simulink model "lookuptable3D"  (Simulink 7.8)
settings: Solver=FixedStepDiscrete  StartTime=0.0  StopTime=10.0  FixedStep=1  RelTol=1e-3
settings Model: Creator=hnine  LastModifiedBy=meta
settings GRTTargetCC: CombineOutputUpdateFcns=on

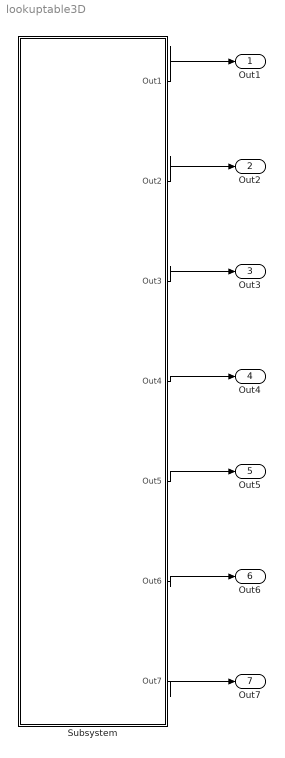
== system lookuptable3D ==
  Subsystem : Subsystem
  Out1 : Outport
  Out2 : Outport  Port=2
  Out3 : Outport  Port=3
  Out4 : Outport  Port=4
  Out5 : Outport  Port=5
  Out6 : Outport  Port=6
  Out7 : Outport  Port=7
  wires:
  Subsystem/1(Out1) -> Out1/1
  Subsystem/2(Out2) -> Out2/1
  Subsystem/3(Out3) -> Out3/1
  Subsystem/7(Out7) -> Out7/1
  Subsystem/4(Out4) -> Out4/1
  Subsystem/5(Out5) -> Out5/1
  Subsystem/6(Out6) -> Out6/1

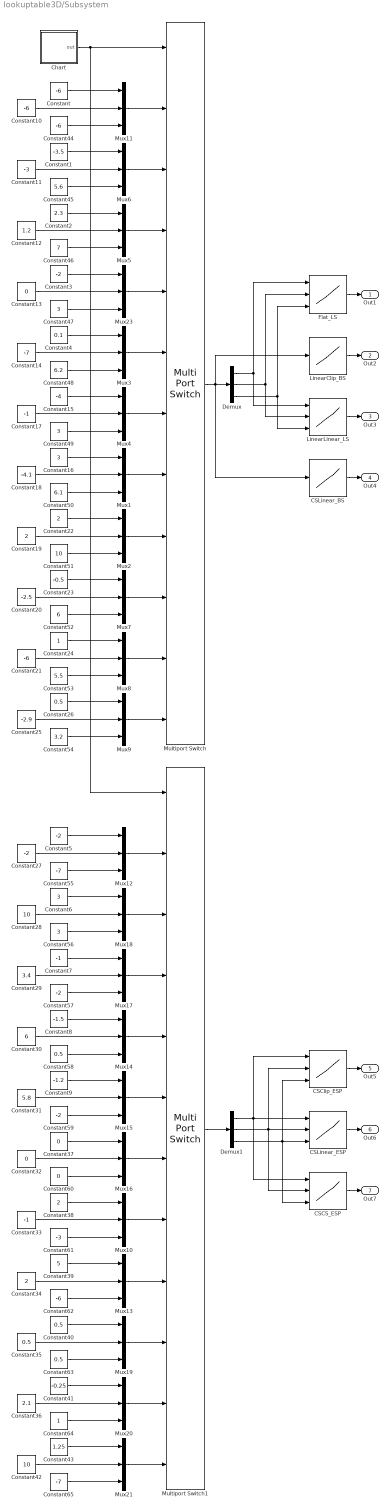
== system lookuptable3D/Subsystem ==
  CSCS_ESP : Lookup_n-D  NumberOfTableDimensions=3  BreakpointsForDimension1=[ -1.5 -0.5 0.5 1.5 ]  BreakpointsForDimension2=[ 0 3 6 9 ]  BreakpointsForDimension3=[ -4 -2.5 -1 0.5 ]  IndexSearchMethod=Evenly spaced points  Table=reshape( [ 10 3.4 1.2 -7 8 -4.5 -4.3 -20 6 9.8 2.1 6.2 4 25 2.4 51 1 -2 2.3 -2 3 -1.4 20 -10 5 2.71 6.667 2.1 7 -25 9.1 -2 9 17 3.4 -1.6 7 -3.3 -1 -15.5 5 3.14 -10 -5.6 3 25 7.33 33 2 6 4.3 8 4 -1.4 4.56 50 6 0 -17 17 8 -25 9.0 -3 ], [ 4 4 4 ] )  InterpMethod=Cubic spline  ExtrapMethod=Cubic spline  RndMeth=Simplest  InputSameDT=on
  CSClip_ESP : Lookup_n-D  NumberOfTableDimensions=3  BreakpointsForDimension1=[ -1.5 -0.5 0.5 1.5 ]  BreakpointsForDimension2=[ 0 3 6 9 ]  BreakpointsForDimension3=[ -4 -2.5 -1 0.5 ]  IndexSearchMethod=Evenly spaced points  Table=reshape( [ 10 3.4 1.2 -7 8 -4.5 -4.3 -20 6 9.8 2.1 6.2 4 25 2.4 51 1 -2 2.3 -2 3 -1.4 20 -10 5 2.71 6.667 2.1 7 -25 9.1 -2 9 17 3.4 -1.6 7 -3.3 -1 -15.5 5 3.14 -10 -5.6 3 25 7.33 33 2 6 4.3 8 4 -1.4 4.56 50 6 0 -17 17 8 -25 9.0 -3 ], [ 4 4 4 ] )  InterpMethod=Cubic spline  ExtrapMethod=Clip  RndMeth=Simplest  InputSameDT=on
  CSLinear_BS : Lookup_n-D  NumberOfTableDimensions=3  BreakpointsForDimension1=[ -4 -2 -0.5 .75 ]  BreakpointsForDimension2=[ -5 -3 -2.5 0 ]  BreakpointsForDimension3=[ 3 5 6 6.2 ]  UseOneInputPortForAllInputData=on  Table=reshape( [ 10 3.4 1.2 -7 8 -4.5 -4.3 -20 6 9.8 2.1 6.2 4 25 2.4 51 1 -2 2.3 -2 3 -1.4 20 -10 5 2.71 6.667 2.1 7 -25 9.1 -2 9 17 3.4 -1.6 7 -3.3 -1 -15.5 5 3.14 -10 -5.6 3 25 7.33 33 2 6 4.3 8 4 -1.4 4.56 50 6 0 -17 17 8 -25 9.0 -3 ], [ 4 4 4 ] )  InterpMethod=Cubic spline  RndMeth=Simplest  InputSameDT=on
  CSLinear_ESP : Lookup_n-D  NumberOfTableDimensions=3  BreakpointsForDimension1=[ -1.5 -0.5 0.5 1.5 ]  BreakpointsForDimension2=[ 0 3 6 9 ]  BreakpointsForDimension3=[ -4 -2.5 -1 0.5 ]  IndexSearchMethod=Linear search  Table=reshape( [ 10 3.4 1.2 -7 8 -4.5 -4.3 -20 6 9.8 2.1 6.2 4 25 2.4 51 1 -2 2.3 -2 3 -1.4 20 -10 5 2.71 6.667 2.1 7 -25 9.1 -2 9 17 3.4 -1.6 7 -3.3 -1 -15.5 5 3.14 -10 -5.6 3 25 7.33 33 2 6 4.3 8 4 -1.4 4.56 50 6 0 -17 17 8 -25 9.0 -3 ], [ 4 4 4 ] )  InterpMethod=Cubic spline  RndMeth=Simplest  InputSameDT=on
  Chart : Stateflow chart  TreatAsAtomicUnit=on
  Constant{,10,21,44,62} (5 alike) : Constant  Value=-6
  Constant1 : Constant  Value=-3.5
  Constant11 : Constant  Value=-3
  Constant12 : Constant  Value=1.2
  Constant{13,32,37,60} (4 alike) : Constant  Value=0
  Constant14 : Constant  Value=-7
  Constant15 : Constant  Value=-4
  Constant{6,16,47,49,56} (5 alike) : Constant  Value=3
  Constant17 : Constant  Value=-1
  Constant18 : Constant  Value=-4.1
  Constant{19,22,34,38} (4 alike) : Constant  Value=2
  Constant2 : Constant  Value=2.3
  Constant20 : Constant  Value=-2.5
  Constant23 : Constant  Value=-0.5
  Constant24 : Constant
  Constant25 : Constant  Value=-2.9
  Constant{26,35,40,58,63} (5 alike) : Constant  Value=0.5
  Constant{3,5,27,57,59} (5 alike) : Constant  Value=-2
  Constant28 : Constant  Value=10
  Constant29 : Constant  Value=3.4
  Constant30 : Constant  Value=6
  Constant31 : Constant  Value=5.8
  Constant33 : Constant  Value=-1
  Constant36 : Constant  Value=2.1
  Constant39 : Constant  Value=5
  Constant4 : Constant  Value=0.1
  Constant41 : Constant  Value=-0.25
  Constant42 : Constant  Value=10
  Constant43 : Constant  Value=1.25
  Constant45 : Constant  Value=5.6
  Constant46 : Constant  Value=7
  Constant48 : Constant  Value=6.2
  Constant50 : Constant  Value=6.1
  Constant51 : Constant  Value=10
  Constant52 : Constant  Value=6
  Constant53 : Constant  Value=5.5
  Constant54 : Constant  Value=3.2
  Constant55 : Constant  Value=-7
  Constant61 : Constant  Value=-3
  Constant64 : Constant
  Constant65 : Constant  Value=-7
  Constant7 : Constant  Value=-1
  Constant8 : Constant  Value=-1.5
  Constant9 : Constant  Value=-1.2
  Demux : Demux  Outputs=3
  Demux1 : Demux  Outputs=3
  Flat_LS : Lookup_n-D  NumberOfTableDimensions=3  BreakpointsForDimension1=[ -4 -2 -0.5 .75 ]  BreakpointsForDimension2=[ -5 -3 -2.5 0 ]  BreakpointsForDimension3=[ 3 5 6 6.2 ]  IndexSearchMethod=Linear search  Table=reshape( [ 10 3.4 1.2 -7 8 -4.5 -4.3 -20 6 9.8 2.1 6.2 4 25 2.4 51 1 -2 2.3 -2 3 -1.4 20 -10 5 2.71 6.667 2.1 7 -25 9.1 -2 9 17 3.4 -1.6 7 -3.3 -1 -15.5 5 3.14 -10 -5.6 3 25 7.33 33 2 6 4.3 8 4 -1.4 4.56 50 6 0 -17 17 8 -25 9.0 -3 ], [ 4 4 4 ] )  InterpMethod=Flat  RndMeth=Simplest  InputSameDT=on
  LinearClip_BS : Lookup_n-D  NumberOfTableDimensions=3  BreakpointsForDimension1=[ -4 -2 -0.5 .75 ]  BreakpointsForDimension2=[ -5 -3 -2.5 0 ]  BreakpointsForDimension3=[ 3 5 6 6.2 ]  UseOneInputPortForAllInputData=on  Table=reshape( [ 10 3.4 1.2 -7 8 -4.5 -4.3 -20 6 9.8 2.1 6.2 4 25 2.4 51 1 -2 2.3 -2 3 -1.4 20 -10 5 2.71 6.667 2.1 7 -25 9.1 -2 9 17 3.4 -1.6 7 -3.3 -1 -15.5 5 3.14 -10 -5.6 3 25 7.33 33 2 6 4.3 8 4 -1.4 4.56 50 6 0 -17 17 8 -25 9.0 -3 ], [ 4 4 4 ] )  ExtrapMethod=Clip  RndMeth=Simplest  InputSameDT=on
  LinearLinear_LS : Lookup_n-D  NumberOfTableDimensions=3  BreakpointsForDimension1=[ -4 -2 -0.5 .75 ]  BreakpointsForDimension2=[ -5 -3 -2.5 0 ]  BreakpointsForDimension3=[ 3 5 6 6.2 ]  IndexSearchMethod=Linear search  Table=reshape( [ 10 3.4 1.2 -7 8 -4.5 -4.3 -20 6 9.8 2.1 6.2 4 25 2.4 51 1 -2 2.3 -2 3 -1.4 20 -10 5 2.71 6.667 2.1 7 -25 9.1 -2 9 17 3.4 -1.6 7 -3.3 -1 -15.5 5 3.14 -10 -5.6 3 25 7.33 33 2 6 4.3 8 4 -1.4 4.56 50 6 0 -17 17 8 -25 9.0 -3 ], [ 4 4 4 ] )  RndMeth=Simplest  InputSameDT=on
  Multiport Switch : MultiPortSwitch  DataPortOrder=Zero-based contiguous  Inputs=11  DiagnosticForDefault=None  zeroidx=on
  Multiport Switch1 : MultiPortSwitch  DataPortOrder=Zero-based contiguous  Inputs=11  DiagnosticForDefault=None  zeroidx=on
  Mux{1..21,23} (22 alike) : Mux  Inputs=3
  Out1 : Outport
  Out2 : Outport  Port=2
  Out3 : Outport  Port=3
  Out4 : Outport  Port=4
  Out5 : Outport  Port=5
  Out6 : Outport  Port=6
  Out7 : Outport  Port=7
  wires:
  Chart/1(out) -> Multiport Switch/1, Multiport Switch1/1
  Constant/1 -> Mux11/1
  Constant1/1 -> Mux6/1
  Constant2/1 -> Mux5/1
  Constant3/1 -> Mux23/1
  Constant4/1 -> Mux3/1
  Mux11/1 -> Multiport Switch/2
  Mux6/1 -> Multiport Switch/3
  Mux5/1 -> Multiport Switch/4
  Mux23/1 -> Multiport Switch/5
  Mux3/1 -> Multiport Switch/6
  Mux4/1 -> Multiport Switch/7
  Mux1/1 -> Multiport Switch/8
  Mux2/1 -> Multiport Switch/9
  Mux7/1 -> Multiport Switch/10
  Mux8/1 -> Multiport Switch/11
  Mux9/1 -> Multiport Switch/12
  Multiport Switch/1 -> LinearClip_BS/1, CSLinear_BS/1, Demux/1
  Demux/1 -> Flat_LS/1, LinearLinear_LS/1
  Demux/2 -> Flat_LS/2, LinearLinear_LS/2
  Constant10/1 -> Mux11/2
  Constant11/1 -> Mux6/2
  Constant12/1 -> Mux5/2
  Constant13/1 -> Mux23/2
  Constant14/1 -> Mux3/2
  Constant15/1 -> Mux4/1
  Constant16/1 -> Mux1/1
  Constant22/1 -> Mux2/1
  Constant23/1 -> Mux7/1
  Constant24/1 -> Mux8/1
  Constant17/1 -> Mux4/2
  Constant18/1 -> Mux1/2
  Constant19/1 -> Mux2/2
  Constant20/1 -> Mux7/2
  Constant21/1 -> Mux8/2
  Constant26/1 -> Mux9/1
  Constant25/1 -> Mux9/2
  Multiport Switch1/1 -> Demux1/1
  Demux1/1 -> CSClip_ESP/1, CSLinear_ESP/1, CSCS_ESP/1
  Demux1/2 -> CSClip_ESP/2, CSLinear_ESP/2, CSCS_ESP/2
  Constant5/1 -> Mux12/1
  Constant6/1 -> Mux18/1
  Constant7/1 -> Mux17/1
  Constant8/1 -> Mux14/1
  Constant9/1 -> Mux15/1
  Constant27/1 -> Mux12/2
  Constant28/1 -> Mux18/2
  Constant29/1 -> Mux17/2
  Constant30/1 -> Mux14/2
  Constant31/1 -> Mux15/2
  Constant37/1 -> Mux16/1
  Constant38/1 -> Mux10/1
  Constant39/1 -> Mux13/1
  Constant40/1 -> Mux19/1
  Constant41/1 -> Mux20/1
  Constant32/1 -> Mux16/2
  Constant33/1 -> Mux10/2
  Constant34/1 -> Mux13/2
  Constant35/1 -> Mux19/2
  Constant36/1 -> Mux20/2
  Constant42/1 -> Mux21/2
  Constant43/1 -> Mux21/1
  Demux/3 -> Flat_LS/3, LinearLinear_LS/3
  Mux12/1 -> Multiport Switch1/2
  Mux18/1 -> Multiport Switch1/3
  Mux17/1 -> Multiport Switch1/4
  Mux14/1 -> Multiport Switch1/5
  Mux15/1 -> Multiport Switch1/6
  Mux16/1 -> Multiport Switch1/7
  Mux10/1 -> Multiport Switch1/8
  Mux13/1 -> Multiport Switch1/9
  Mux19/1 -> Multiport Switch1/10
  Mux20/1 -> Multiport Switch1/11
  Mux21/1 -> Multiport Switch1/12
  Constant44/1 -> Mux11/3
  Constant45/1 -> Mux6/3
  Constant46/1 -> Mux5/3
  Constant47/1 -> Mux23/3
  Constant48/1 -> Mux3/3
  Constant49/1 -> Mux4/3
  Constant50/1 -> Mux1/3
  Constant51/1 -> Mux2/3
  Constant52/1 -> Mux7/3
  Constant53/1 -> Mux8/3
  Constant54/1 -> Mux9/3
  Demux1/3 -> CSLinear_ESP/3, CSClip_ESP/3, CSCS_ESP/3
  Constant55/1 -> Mux12/3
  Constant56/1 -> Mux18/3
  Constant57/1 -> Mux17/3
  Constant58/1 -> Mux14/3
  Constant59/1 -> Mux15/3
  Constant60/1 -> Mux16/3
  Constant61/1 -> Mux10/3
  Constant62/1 -> Mux13/3
  Constant63/1 -> Mux19/3
  Constant64/1 -> Mux20/3
  Constant65/1 -> Mux21/3
  Flat_LS/1 -> Out1/1
  LinearClip_BS/1 -> Out2/1
  LinearLinear_LS/1 -> Out3/1
  CSLinear_BS/1 -> Out4/1
  CSClip_ESP/1 -> Out5/1
  CSLinear_ESP/1 -> Out6/1
  CSCS_ESP/1 -> Out7/1

== stateflow chart Subsystem/Chart ==
  state count
    en: out = 0;
    du: out = out + 1;
  (default) -> count
  count -> count : [ out >= 10 ]
  data: out output double =0
